simulink model "mfiletest"  (Simulink 7.7)
settings: Solver=FixedStepDiscrete  StartTime=0.0  StopTime=10.0  FixedStep=1  RelTol=1e-3
settings Model: Creator=hnine  LastModifiedBy=hnine
settings DataIOCC: SaveFormat=Structure

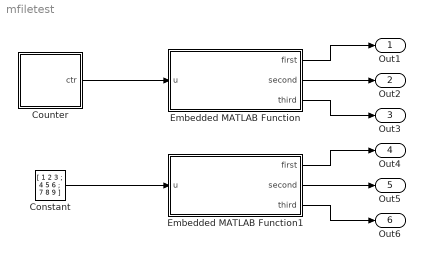
== system mfiletest ==
  Constant : Constant  Value=[ 1 2 3 ; 4 5 6 ; 7 8 9 ]
  Counter : Stateflow chart  TreatAsAtomicUnit=on
  Embedded MATLAB Function : Stateflow chart  TreatAsAtomicUnit=on
  Embedded MATLAB Function1 : Stateflow chart  TreatAsAtomicUnit=on
  Out1 : Outport
  Out2 : Outport  Port=2
  Out3 : Outport  Port=3
  Out4 : Outport  Port=4
  Out5 : Outport  Port=5
  Out6 : Outport  Port=6
  wires:
  Counter/1(ctr) -> Embedded MATLAB Function/1(u)
  Embedded MATLAB Function/1(first) -> Out1/1
  Embedded MATLAB Function/2(second) -> Out2/1
  Embedded MATLAB Function/3(third) -> Out3/1
  Constant/1 -> Embedded MATLAB Function1/1(u)
  Embedded MATLAB Function1/1(first) -> Out4/1
  Embedded MATLAB Function1/2(second) -> Out5/1
  Embedded MATLAB Function1/3(third) -> Out6/1

== stateflow chart Counter ==
  state s1
  (default) -> s1
  s1 -> s1 [order 1] : [ctr < 4] / ctr = ctr+1;
  s1 -> s1 [order 2] : [ctr >= 4] / ctr = -2;
  data: ctr output double =1

== matlab function Embedded MATLAB Function ==
  data: u input double; first output double; second output double; third output double
function [first,second,third] = fcn(u)
%#eml

[first,second,third]=multiply(u, 1, 2, 3);

== matlab function Embedded MATLAB Function1 ==
  data: u input double; first output double; second output double; third output double
function [first,second,third] = fcn(u)
%#eml

[first,second,third]=multiply(u, 4, 5, 6);
